simulink model "sim_trot_d_bo"  (R2025b)
settings: Solver=VariableStepAuto  StartTime=0.0  StopTime=t_sim  MaxStep=Te/100  RelTol=1e-3
undefined symbols (not defined in the file): C14, C2, C5, K, Kh, Ki, L, R, R5, R6, R7, Si, Te
settings Model: Creator=thibaut  LastModifiedBy=thibaut

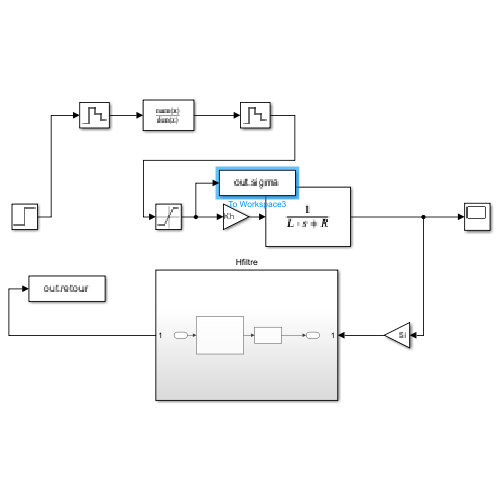
[thumbnail: Simulink's stored preview of the top-level diagram]
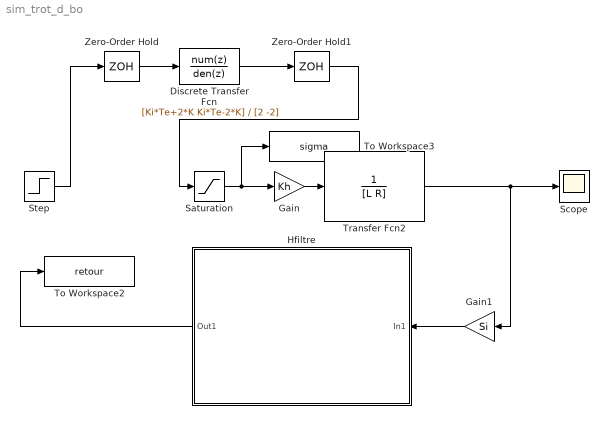
== system sim_trot_d_bo ==
  Discrete Transfer Fcn : DiscreteTransferFcn  Numerator=[Ki*Te+2*K Ki*Te-2*K]  Denominator=[2 -2]
  Gain : Gain  Gain=Kh
  Gain1 : Gain  Gain=Si
  Hfiltre : Subsystem
  Saturation : Saturate  UpperLimit=0.495  LowerLimit=-0.495
  Scope : Scope
      settings: ActiveDisplayYMinimum=-56.003937909430292  ActiveDisplayYMaximum=73.44419626682577
  Step : Step  Time=0  After=0.1  SampleTime=0
  To Workspace2 : ToWorkspace  VariableName=retour  SaveFormat=Timeseries  SampleTime=-1
  To Workspace3 : ToWorkspace  VariableName=sigma  SaveFormat=Timeseries  SampleTime=-1
  Transfer Fcn2 : TransferFcn  Denominator=[L R]
  Zero-Order Hold : ZeroOrderHold  SampleTime=Te
  Zero-Order Hold1 : ZeroOrderHold  SampleTime=Te
  wires:
  Step/1 -> Zero-Order Hold/1
  Gain/1 -> Transfer Fcn2/1
  Transfer Fcn2/1 -> Scope/1, Gain1/1
  Gain1/1 -> Hfiltre/1(In1)
  Hfiltre/1(Out1) -> To Workspace2/1
  Zero-Order Hold/1 -> Discrete Transfer Fcn/1
  Discrete Transfer Fcn/1 -> Zero-Order Hold1/1
  Saturation/1 -> To Workspace3/1, Gain/1
  Zero-Order Hold1/1 -> Saturation/1

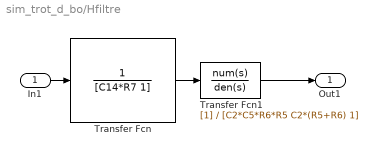
== system sim_trot_d_bo/Hfiltre ==
  In1 : Inport
  Transfer Fcn : TransferFcn  Denominator=[C14*R7 1]
  Transfer Fcn1 : TransferFcn  Denominator=[C2*C5*R6*R5 C2*(R5+R6) 1]
  Out1 : Outport
  wires:
  In1/1 -> Transfer Fcn/1
  Transfer Fcn/1 -> Transfer Fcn1/1
  Transfer Fcn1/1 -> Out1/1
